simulink model "szybkozmienny_dyskr2"  (R2017b)
settings: Solver=FixedStepDiscrete  StartTime=0.0  StopTime=0.0  RelTol=1e-3
libraries: CPOiS_SourcesSinks x8, CPOiS_DataManipulation x3
settings Model: Creator=alis  LastModifiedBy=alis

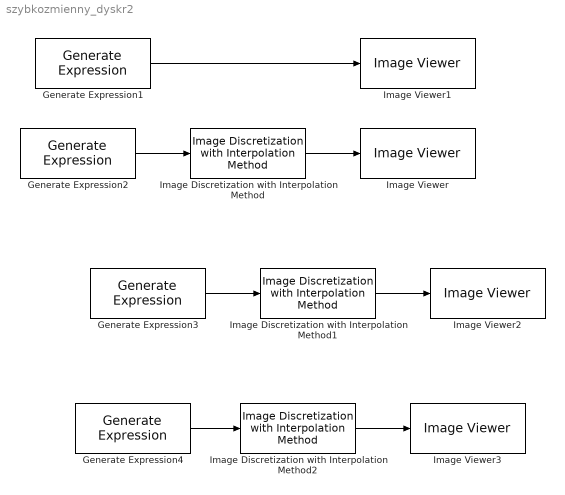
== system szybkozmienny_dyskr2 ==
  Generate Expression{1..4} (4 alike) : CPOiS_SourcesSinks/Generate Expression  Width=256  Height=256  Expression=255.*(mod(W,4)>1)
      settings: SourceProductName=CPOiS - Digital image and signal processing
  Image Discretization with Interpolation Method : CPOiS_DataManipulation/Image Discretization with Interpolation Method  factor=3  method=nearest
      settings: SourceProductName=CPOiS - Digital image and signal processing
  Image Discretization with Interpolation Method1 : CPOiS_DataManipulation/Image Discretization with Interpolation Method  factor=3  method=bilinear
      settings: SourceProductName=CPOiS - Digital image and signal processing
  Image Discretization with Interpolation Method2 : CPOiS_DataManipulation/Image Discretization with Interpolation Method  factor=3  method=bicubic
      settings: SourceProductName=CPOiS - Digital image and signal processing
  Image Viewer{,1..3} (4 alike) : CPOiS_SourcesSinks/Image Viewer
      settings: SourceProductName=CPOiS - Digital image and signal processing
  wires:
  Generate Expression3/1 -> Image Discretization with Interpolation Method1/1
  Generate Expression1/1 -> Image Viewer1/1
  Image Discretization with Interpolation Method/1 -> Image Viewer/1
  Generate Expression2/1 -> Image Discretization with Interpolation Method/1
  Generate Expression4/1 -> Image Discretization with Interpolation Method2/1
  Image Discretization with Interpolation Method2/1 -> Image Viewer3/1
  Image Discretization with Interpolation Method1/1 -> Image Viewer2/1
